simulink library "NCS_Library"  (R2019a)
settings: Solver=VariableStepAuto  StartTime=0.0  StopTime=10.0  RelTol=1e-3
values from neighbouring files (symbols this model uses):
  A = 10    [Parameter.m]
  band = 100000000    [Parameter.m]
  BER = 0    [Parameter.m]
  c = 5000000    [Parameter.m]
  c1 = 4.33    [Parameter.m]
  c2 = 3.16    [Parameter.m]
  CAN2EthernetDelay = 0.000    (= 0)    [Parameter.m]
  cR = 1.5*10^-3    (= 0.0015)    [Parameter.m]
  cw = (cwE * 2 + cwM * (nW_ges-2))/nW_ges    (= 0.1475)    [Parameter.m]
  cwE = 0.35    [Parameter.m]
  cwM = 0.08    [Parameter.m]
  Cycle_Controller = 0    [Parameter.m]
  CyclePLC = 24/1000    (= 0.024)    [Parameter.m]
  d = 800000    [Parameter.m]
  Dr = 0.92    [Parameter.m]
  Ethernet2CANDelay = 0.005    [Parameter.m]
  F_konst = 70892    [Parameter.m]
  FA = 100000    [Parameter.m]
  FB_WB_max = 10000    [Parameter.m]
  FBel_an = iG*nG*F_KZmax*nBan*R_mR/(Dr/2)    (= 28197.4297239)    [Parameter.m]
  FBel_frei = iG*nG*F_KZmax*nBfrei*R_mW/(Dr/2)    (= 29270.6882948)    [Parameter.m]
  Fmaxdyn = 300000    [Parameter.m]
  g = 9.81    [Parameter.m]
  i = 0    [Parameter.m]
  J = 1/2*mA*(Dr/2)^2    (= 158.7)    [Parameter.m]
  k1 = 0.095    [Parameter.m]
  k2 = 9.26/3.6    (= 2.57222222222)    [Parameter.m]
  k3 = 4.63/3.6    (= 1.28611111111)    [Parameter.m]
  mges = 58000    [Parameter.m]
  mu = [mu1 mu2]    [Parameter.m]
  muBel1 = 0.42    [Parameter.m]
  muBel2 = 0.36    [Parameter.m]
  n = 0.001    [Parameter.m]
  n_Mg = 4    [Parameter.m]
  n_WB = 4    [Parameter.m]
  nA = 4    [Parameter.m]
  nBan = 2    [Parameter.m]
  nBfrei = 3    [Parameter.m]
  nM = 4    [Parameter.m]
  nW_an = 4    [Parameter.m]
  P_max = 8200000    [Parameter.m]
  Q = 10    [Parameter.m]
  r_reib = 600    [Parameter.m]
  rho = 1.08    [Parameter.m]
  rhoL = 1.225    [Parameter.m]
  Size = 8    [Parameter.m]
  slip = [s1 s2]    [Parameter.m]
  tol = 0.05    [Parameter.m]
  v00 = 100/3.6    (= 27.7777777778)    [Parameter.m]
  v_grenz = 60/3.6    (= 16.6666666667)    [Parameter.m]
  v_opt = 75/3.6    (= 20.8333333333)    [Parameter.m]
  W_opt = 0.5    [Parameter.m]
  WB = 1    [Parameter.m]
  y_opt = sqrt(W_opt)/((1+sqrt(W_opt))^2+W_opt)    [Parameter.m]
undefined symbols (not defined in the file or in its folder): BUSCapacity, CableLength, controlGate, D_dyn, D_mg, EnableBurst, EnableToF, entity, Entity_out, Gate, Gate_4, Gate_5, Gate_ACK, Gate_copy, Gate_RX, getData, gettime, I_dyn, I_mg, m, magnitude, P_dyn, P_mg, ReadAttributes, readdata, ReadData, ReadSize, sigbuilder_block, Timeout, ToB, ToF, v0, v_d, v_soll
libraries: simulink x176, $bdroot x102
(part 9 of 12)

== system NCS_Library/Network/ETB/Subsystem2/Routing Table/Get Routing Table ==
  note: Compute RT
  note: Receive Data
  note: Send Data
  RouterID : Inport
  s1 : Inport  Port=2
  s2 : Inport  Port=3
  s3 : Inport  Port=4
  Failed : Inport  Port=5
  Compute Routing Table : Subsystem
  Compute routing matrix RM : Subsystem
  Constant1 : Constant
  Constant2 : Constant
  Delay : Delay  DelayLength=1
  Delay1 : Delay  DelayLength=1
  Detect Change : simulink/Logic and Bit Operations/Detect Change  vinit=0  OutDataTypeStr=boolean
  Display : Display
  Entity Gate : EntityGate  InputPortMessageModes=m,m  OutputPortMessageModes=m  OperatingMode=Release gate  OpenGateAtSimulationStart=on
  Entity Generator : EntityGenerator  InputPortMessageModes=m  OutputPortMessageModes=m  GenerationMethod=Event-based  Period=0.5  GenerateAction=[entity.R_local] = writedata();  AttributeName=ID|S1|S2|S3|S4|S5  AttributeInitialValue=1|0|0|0|0|0  EntityType=Bus object  EntityTypeName=Router
      settings: InputPortMap=u0
  Entity Multicast : EntityMulticast  InputPortMessageModes=m  MulticastTag=Router
  Entity Terminator : EntityTerminator  InputPortMessageModes=m  EntryAction=readdata(entity.R_local);  NumberEntitiesArrived=on
      settings: OutputPortMap=o0
  Failed1 : InportShadow  Port=5
  Ground : Ground
  Ground1 : Ground
  Message Send : MessageSend  OutputPortMessageModes=m  ShowEnablePort=on
      settings: InputPortMap=e0,u1
  Message Send1 : MessageSend  OutputPortMessageModes=m  ShowEnablePort=on
      settings: InputPortMap=e0,u1
  Multicast Receive Queue : EntityQueue  OutputPortMessageModes=m  Capacity=50  EntityArrivalSource=Multicast  MulticastTag=Router
      settings: OutputPortMap=o5
  Router Control : Stateflow chart  TreatAsAtomicUnit=on
  RouterID1 : InportShadow
  Simulink Function1 : Subsystem  TreatAsAtomicUnit=on
  Simulink Function2 : Subsystem  TreatAsAtomicUnit=on
  RT : Outport
  FIN : Outport  Port=2
  wires:
  Compute routing matrix RM/2(RM_global) -> Compute Routing Table/2(RM)
  Simulink Function2/1(RM_in) -> Compute routing matrix RM/1(RM_in)
  Compute Routing Table/1(FIN_Init) -> FIN/1, Delay1/1
  RouterID1/1 -> Compute Routing Table/1(ID)
  Message Send/1 -> Entity Gate/1
  Multicast Receive Queue/1 -> Entity Gate/2
  Delay/1 -> Message Send/1
  Detect Change/1 -> Delay/1
  Entity Terminator/1 -> Detect Change/1
  Constant1/1 -> Message Send/2
  Entity Gate/1 -> Entity Terminator/1
  Message Send1/1 -> Entity Generator/1
  Entity Generator/1 -> Entity Multicast/1
  RouterID/1 -> Simulink Function1/1(In1)
  s1/1 -> Simulink Function1/2(s1)
  s2/1 -> Simulink Function1/3(In8)
  s3/1 -> Simulink Function1/4(In9)
  Ground/1 -> Simulink Function1/5(In10)
  Ground1/1 -> Simulink Function1/6(In11)
  Constant2/1 -> Message Send1/2
  Simulink Function2/2(Refresh) -> Router Control/1(Refresh)
  Router Control/2(Init) -> Compute routing matrix RM/Enable
  Router Control/1(Tx) -> Display/1, Message Send1/1
  Compute Routing Table/2(RT) -> RT/1
  Failed/1 -> Simulink Function1/7(Failed)
  Failed1/1 -> Router Control/2(Failed)
  Delay1/1 -> Router Control/3(FIN)
  Compute routing matrix RM/1(FIN_RM) -> Compute Routing Table/Enable

== system NCS_Library/Network/ETB/Subsystem2/Routing Table/Subsystem ==
  Clock : Clock
  Compare To Constant : simulink/Logic and Bit Operations/Compare To Constant  relop=>=  const=ToF  OutDataTypeStr=uint8
  Constant3 : Constant  Value=EnableToF
  Display2 : Display
  Display3 : Display
  Logical Operator : Logic  AllPortsSameDT=off  OutDataTypeStr=boolean
  Out1 : Outport
  wires:
  Compare To Constant/1 -> Logical Operator/1, Display3/1
  Constant3/1 -> Logical Operator/2, Display2/1
  Clock/1 -> Compare To Constant/1
  Logical Operator/1 -> Out1/1

== system NCS_Library/Network/Gateway/Gateway1/CAN Interface/CAN Interface ==
  note: Receiver
  note: Transmitter
  d_in : Inport
  Current Message : EntityQueue  InputPortMessageModes=m  OutputPortMessageModes=m  Capacity=2  EntryAction=controlGate(0);  ExitAction=controlGate(1);
      settings: OutputPortMap=o5
  Damaged Message : EntityTerminator  InputPortMessageModes=m  NumberEntitiesArrived=on
      settings: OutputPortMap=o0
  Display{,1..3} (4 alike) : Display
  Drop Dated Message upon Buffer Overflow : EntityOutputSwitch  InputPortMessageModes=m  OutputPortMessageModes=m,m  SwitchAttributeName=Attribute1
  Entity Replicator : EntityReplicator  InputPortMessageModes=m  OutputPortMessageModes=m,m
  Entity Replicator1 : EntityReplicator  InputPortMessageModes=m  OutputPortMessageModes=m,m
  Entity Terminator : EntityTerminator  InputPortMessageModes=m
  Failure Control CAN : $bdroot/Network/Applications/Failure Control CAN  SystemSampleTime=-1
  Failure Control CAN1 : $bdroot/Network/Applications/Failure Control CAN  SystemSampleTime=-1
  Message Release Control : EntityGate  InputPortMessageModes=m,m  OutputPortMessageModes=m  OpenGateAtSimulationStart=on
  Message from Bus : EntityQueue  OutputPortMessageModes=m  Capacity=20  EntityArrivalSource=Multicast  MulticastTag=FromBus_1
      settings: OutputPortMap=o5
  Path Combiner : EntityInputSwitch  InputPortMessageModes=m,m  OutputPortMessageModes=m
  Re-Transmission Control : Subsystem
  Received Message : EntityServer  InputPortMessageModes=m  OutputPortMessageModes=m  Capacity=1  ServiceTimeValue=0
  Reception Control : Stateflow chart  TreatAsAtomicUnit=on
  Replicate for Re-Transmission : EntityReplicator  InputPortMessageModes=m  OutputPortMessageModes=m,m,m  NumberReplicas=2
      settings: OutputPortMap=o0,o1,o2
  Send Message to Bus : EntityMulticast  InputPortMessageModes=m  MulticastTag=ToBus_1
  Signal To CAN Message : Subsystem
  Simulink Function : Subsystem  TreatAsAtomicUnit=on
  Sort : EntityOutputSwitch  InputPortMessageModes=m,m  OutputPortMessageModes=m,m,m  NumberOutputPorts=3  SwitchingCriterion=From control port  SwitchAttributeName=Attribute1
      settings: InputPortMap=u0,u1  OutputPortMap=o0,o1,o2
  Subscribed Message : EntityTerminator  InputPortMessageModes=m  NumberEntitiesArrived=on
      settings: OutputPortMap=o0
  Transmission Buffer : EntityQueue  InputPortMessageModes=m  OutputPortMessageModes=m  Capacity=15  QueueType=Priority  PrioritySource=ID
      settings: OutputPortMap=o5
  Unsubscribed Message : EntityTerminator  InputPortMessageModes=m  NumberEntitiesArrived=on
      settings: OutputPortMap=o0
  CAN_Message : Outport
  wires:
  Sort/1 -> Entity Replicator1/1
  Failure Control CAN/1 -> Message Release Control/2
  Replicate for Re-Transmission/3 -> Reception Control/1(TX)
  Simulink Function/1(ctrl) -> Message Release Control/1
  Current Message/1 -> Re-Transmission Control/1(IN)
  Reception Control/3(ReTX) -> [ReTX]
  Transmission Buffer/1 -> Failure Control CAN/1
  Re-Transmission Control/1(OUT) -> Drop Dated Message upon Buffer Overflow/1
  Message from Bus/1 -> Failure Control CAN1/1
  Entity Replicator/1 -> Reception Control/2(RX)
  Replicate for Re-Transmission/2 -> Send Message to Bus/1
  Failure Control CAN1/1 -> Entity Replicator/1
  Unsubscribed Message/1 -> Display1/1
  Drop Dated Message upon Buffer Overflow/2 -> Entity Terminator/1
  Path Combiner/1 -> Transmission Buffer/1
  Replicate for Re-Transmission/1 -> Current Message/1
  Damaged Message/1 -> Display/1
  [Reset] -> Re-Transmission Control/3(Reset)
  Re-Transmission Control/2(#TX) -> Display3/1
  d_in/1 -> Signal To CAN Message/1(Data)
  Signal To CAN Message/1(MsgOut) -> Path Combiner/2
  Entity Replicator/2 -> Received Message/1
  Reception Control/2(Success) -> [Reset]
  Drop Dated Message upon Buffer Overflow/1 -> Path Combiner/1
  Subscribed Message/1 -> Display2/1
  [ReTX] -> Re-Transmission Control/2(ReTX)
  Sort/2 -> Unsubscribed Message/1
  Message Release Control/1 -> Replicate for Re-Transmission/1
  Reception Control/1(Port) -> Sort/1
  Sort/3 -> Damaged Message/1
  Received Message/1 -> Sort/2
  Entity Replicator1/2 -> Subscribed Message/1
  Entity Replicator1/1 -> CAN_Message/1

== system NCS_Library/Network/Gateway/Gateway1/CAN Interface/Entry Control ==
  note: new entity in buffer AND buffer is NOT flushed
  note: refresh
  FLUSH : Inport
  n_packets : Inport  Port=2
  Add : Sum
  Add1 : Sum  Inputs=+-
  Compare To Zero : simulink/Logic and Bit Operations/Compare To Zero  relop===  OutDataTypeStr=boolean
  Compare To Zero1 : simulink/Logic and Bit Operations/Compare To Zero  relop=>  OutDataTypeStr=boolean
  Delay : Delay  DelayLength=1  InitialCondition=1
  Display1 : Display
  Enabled Subsystem : Subsystem  TreatAsAtomicUnit=on
  Entity Server : EntityServer  InputPortMessageModes=m  OutputPortMessageModes=n,m  Capacity=1  ServiceTimeValue=0  NumberEntitiesDeparted=on
      settings: OutputPortMap=o0,o9
  FLUSH1 : InportShadow
  Memory : Memory
  Multiply : Product
  Out1 : Outport
  wires:
  n_packets/1 -> Add1/1, Memory/1
  Memory/1 -> Add1/2
  Add1/1 -> Compare To Zero1/1
  Compare To Zero/1 -> Multiply/1
  Compare To Zero1/1 -> Multiply/2
  Multiply/1 -> Add/1
  FLUSH/1 -> Compare To Zero/1
  Add/1 -> Enabled Subsystem/Enable
  Delay/1 -> Add/2
  FLUSH1/1 -> Delay/1
  Entity Server/1 -> Display1/1
  Entity Server/2 -> Out1/1
  Enabled Subsystem/1(Out1) -> Entity Server/1

== system NCS_Library/Network/Gateway/Gateway1/CAN Interface/Gate Control ==
  note: Time condition
  note: Number condition
  n_packets : Inport
  Add : Sum  Inputs=-+
  Add2 : Sum
  Add3 : Sum  Inputs=-+-+
  Clock : Clock
  Compare To Zero : simulink/Logic and Bit Operations/Compare To Zero  relop=>=  OutDataTypeStr=uint8
  Compare To Zero1 : simulink/Logic and Bit Operations/Compare To Zero  relop=>=  OutDataTypeStr=uint8
  Compare To Zero2 : simulink/Logic and Bit Operations/Compare To Zero  relop=>  OutDataTypeStr=uint8
  Constant : Constant  Value=T_Tx
  Constant1 : Constant  Value=MaxNum
  Constant2 : Constant  Value=1e-10
  Memory : Memory  InheritSampleTime=on
  Multiply : Product
  Multiply1 : Product
  Save last release time1 : Subsystem
  FLUSH : Outport
  wires:
  Compare To Zero2/1 -> Multiply/2
  Multiply/1 -> Save last release time1/Enable, FLUSH/1
  Add2/1 -> Multiply/1
  Compare To Zero/1 -> Add2/2
  n_packets/1 -> Add/2, Compare To Zero2/1
  Constant1/1 -> Add/1
  Compare To Zero1/1 -> Add2/1
  Add/1 -> Compare To Zero/1
  Multiply1/1 -> Add3/1
  Constant/1 -> Multiply1/2, Add3/3  "T_Tx"
  Memory/1 -> Multiply1/1, Save last release time1/1(Time)
  Clock/1 -> Add3/2
  Constant2/1 -> Add3/4  "Compensate numeric drift"
  Save last release time1/1(Out1) -> Memory/1
  Add3/1 -> Compare To Zero1/1

== system NCS_Library/Network/Gateway/Gateway1/CAN Interface/Read Data ==
  ReadData : TriggerPort  TriggerType=function-call  IsSimulinkFunction=on  FunctionName=ReadData  FunctionVisibility=scoped  VariantControl=(inherit)
  SensorType : ArgIn  DisableCoverage=on  OutDataTypeStr=uint8  ArgumentName=SensorType
  SensorType1 : ArgIn  DisableCoverage=on  Port=2  ArgumentName=Data
  Type : Outport
  Data : Outport  Port=2  OutputWhenDisabled=reset  InitialOutput=0
  wires:
  SensorType1/1 -> Data/1
  SensorType/1 -> Type/1

== system NCS_Library/Network/Gateway/Gateway1/CAN Interface/Save Data ==
  Type : Inport
  Data : Inport  Port=2
  FLUSH : Inport  Port=3
  Add : Sum
  Delay : Delay  DelayLength=1  InitialCondition=1
  Detect Change : simulink/Logic and Bit Operations/Detect Change  vinit=0  OutDataTypeStr=boolean
  Detect Change1 : simulink/Logic and Bit Operations/Detect Change  vinit=0  OutDataTypeStr=boolean
  Display : Display
  Display1 : Display
  Display2 : Display
  Hold Data : Stateflow chart  TreatAsAtomicUnit=on
  MATLAB Function : MATLAB Function  TreatAsAtomicUnit=on
  Memory : Memory  InheritSampleTime=on
  OutData : Outport
  wires:
  Detect Change1/1 -> Add/2
  Detect Change/1 -> Add/1
  Add/1 -> MATLAB Function/2(write)
  Memory/1 -> MATLAB Function/5(M_Data_old)
  FLUSH/1 -> Hold Data/1(Flush), Delay/1
  MATLAB Function/1(M_Data) -> Hold Data/2(InData), Memory/1
  Type/1 -> Display2/1, MATLAB Function/3(Type), Detect Change/1
  Data/1 -> Display1/1, MATLAB Function/4(Data), Detect Change1/1
  Delay/1 -> MATLAB Function/1(refresh)
  Hold Data/1(OutData) -> OutData/1, Display/1

== system NCS_Library/Network/Gateway/Gateway1/Ethernet Interface/Enabled Subsystem ==
  In1 : Inport
  Enable : EnablePort
  Out1 : Outport
  wires:
  In1/1 -> Out1/1

== system NCS_Library/Network/Gateway/Gateway1/Ethernet Interface/Protocol Stack ==
  Signal : Inport
  Parameter : Inport  Port=2
  RxFromBus : Inport  Port=3
  Bus Creator1 : BusCreator  Inputs=13
  Bus Selector : BusSelector  OutputSignals=SDTv2,T_Tx,msgType
  CycleRx : EntityServer  InputPortMessageModes=m  OutputPortMessageModes=m  Capacity=inf  ServiceTimeValue=CycleRx
  CycleTx : EntityServer  InputPortMessageModes=m  OutputPortMessageModes=m  Capacity=inf  ServiceTimeValue=CycleTx
  Data Type Conversion{,1..6} (7 alike) : DataTypeConversion  OutDataTypeStr=double
  Detect Change : simulink/Logic and Bit Operations/Detect Change  vinit=0  OutDataTypeStr=boolean
  IP : $bdroot/Network/ETB/OSI Layers/IP  SystemSampleTime=-1
  MAC Controller : $bdroot/Network/ETB/OSI Layers/MAC Controller  SystemSampleTime=-1
  Multiply : Product
  SDTv2 : $bdroot/Network/ETB/OSI Layers/SDTv2  SystemSampleTime=-1
  Signal1 : InportShadow
  TRDP PD : $bdroot/Network/ETB/OSI Layers/TRDP PD  SystemSampleTime=-1
  TRDP Timeout : $bdroot/Network/ETB/OSI Layers/TRDP Timeout  SystemSampleTime=-1
  UDP Single-Port : $bdroot/Network/ETB/OSI Layers/UDP Single-Port  SystemSampleTime=-1
  Data : Outport
  Recorder : Outport  Port=2
  TxToBus : Outport  Port=3
  wires:
  Data Type Conversion6/1 -> Bus Creator1/7  "#Receive"
  Data Type Conversion5/1 -> Bus Creator1/9  "#damaged"
  Data Type Conversion4/1 -> Bus Creator1/12  "Retry"
  Data Type Conversion3/1 -> Bus Creator1/3  "SSC"
  Data Type Conversion2/1 -> Bus Creator1/8  "msgType_receive"
  Data Type Conversion1/1 -> Bus Creator1/5  "#Transmit"
  Bus Selector/1 -> SDTv2/2, [SDTv2]  "<SDTv2>"
  Detect Change/1 -> Data Type Conversion4/1
  MAC Controller/3 -> Detect Change/1  "Retry"
  MAC Controller/4 -> TxToBus/1
  Bus Selector/3 -> SDTv2/4  "<msgType>"
  TRDP PD/1 -> SDTv2/5
  Bus Selector/2 -> SDTv2/3  "<T_Tx>"
  TRDP PD/2 -> SDTv2/6
  SDTv2/4 -> TRDP PD/1
  TRDP PD/7 -> UDP Single-Port/1
  Bus Creator1/1 -> Recorder/1
  Data Type Conversion/1 -> Bus Creator1/6  "msgType_transmit"
  Parameter/1 -> TRDP PD/3, MAC Controller/2, IP/2, Bus Selector/1
  Signal/1 -> SDTv2/1, Bus Creator1/1  "Signal"
  MAC Controller/2 -> Bus Creator1/11  "#collision"
  UDP Single-Port/1 -> TRDP PD/4
  IP/1 -> UDP Single-Port/2
  UDP Single-Port/2 -> IP/1
  RxFromBus/1 -> MAC Controller/3
  [SDTv2] -> Bus Creator1/13  "SDTv2"
  SDTv2/2 -> Data Type Conversion3/1
  SDTv2/3 -> Bus Creator1/4  "Phase"
  TRDP PD/3 -> Data Type Conversion1/1
  TRDP PD/4 -> Data Type Conversion/1
  TRDP PD/5 -> TRDP Timeout/1, Data Type Conversion6/1
  TRDP PD/6 -> Data Type Conversion2/1
  IP/2 -> Data Type Conversion5/1
  IP/3 -> Bus Creator1/10  "delay"
  CycleRx/1 -> IP/3
  MAC Controller/1 -> CycleRx/1
  IP/4 -> CycleTx/1
  CycleTx/1 -> MAC Controller/1
  Signal1/1 -> TRDP PD/2  "Signal"
  Multiply/1 -> Data/1, Bus Creator1/2
  SDTv2/1 -> Multiply/2  "Data"
  [Valid] -> Multiply/1
  TRDP Timeout/1 -> [Valid]

== system NCS_Library/Network/Gateway/Gateway1/Ethernet Interface/Subsystem4 ==
  Data : Inport
  Add3 : Sum  Inputs=-+-+
  Chart : Stateflow chart  TreatAsAtomicUnit=on
  Clock : Clock
  Compare To Zero1 : simulink/Logic and Bit Operations/Compare To Zero  relop=>=  OutDataTypeStr=uint8
  Constant8 : Constant  Value=T_Tx_CAN
  Constant9 : Constant  Value=1e-10
  Detect Change : simulink/Logic and Bit Operations/Detect Change  vinit=0  OutDataTypeStr=boolean
  Display : Display
  Display1 : Display
  Display2 : Display
  MATLAB Function : MATLAB Function  TreatAsAtomicUnit=on
  Memory1 : Memory  InheritSampleTime=on
  Multiply1 : Product
  Save num release : Subsystem
  Push : Outport
  wires:
  Add3/1 -> Compare To Zero1/1
  Constant9/1 -> Add3/4  "Compensate numeric drift"
  Save num release/1(Out1) -> Memory1/1
  Constant8/1 -> Multiply1/2, Add3/3  "T_Tx"
  Memory1/1 -> Save num release/1(Time), Multiply1/1
  Multiply1/1 -> Add3/1
  Clock/1 -> Add3/2
  Data/1 -> Display2/1, Detect Change/1, MATLAB Function/1(Data)
  Chart/1(Push) -> Push/1
  Compare To Zero1/1 -> Save num release/Enable, Display1/1, Chart/1(TIME)
  Detect Change/1 -> MATLAB Function/2(Change)
  MATLAB Function/1(NEW) -> Chart/2(NEW), Display/1

== system NCS_Library/Network/Gateway/Gateway1/Ethernet Interface/User Interface ==
  note: User defined Parameters
  Add : Sum  Inputs=+-
  Bus Creator : BusCreator  Inputs=8
  Constant : Constant  Value=Address  OutDataTypeStr=uint16
  Constant1 : Constant  Value=Destination  OutDataTypeStr=uint16
  Constant2 : Constant  Value=0  OutDataTypeStr=double
  Constant3 : Constant  Value=3  OutDataTypeStr=uint8
  Constant4 : Constant  Value=SDTv2  OutDataTypeStr=double
  Constant5 : Constant
  Constant6 : Constant  Value=Port  OutDataTypeStr=uint16
  Constant7 : Constant  Value=ReplyAddress  OutDataTypeStr=uint16
  MATLAB Function : MATLAB Function  TreatAsAtomicUnit=on
  MATLAB Function1 : MATLAB Function  TreatAsAtomicUnit=on
  Subscribe : Constant  Value=Subscribe  OutDataTypeStr=uint16
  Subsystem1 : Subsystem
  Subsystem2 : Subsystem
  Subsystem3 : Subsystem
  Out1 : Outport
  wires:
  Add/1 -> Bus Creator/8  "SDTv2"
  Subscribe/1 -> MATLAB Function1/1(u)
  Constant6/1 -> Bus Creator/5  "Port"
  MATLAB Function1/1(y) -> Bus Creator/3  "Subscribe"
  Constant4/1 -> Add/1
  Constant/1 -> Subsystem1/1(In1)
  Subsystem1/1(Out1) -> Bus Creator/1  "Address"
  Constant3/1 -> MATLAB Function/1(u)
  Subsystem3/1(Out1) -> Bus Creator/4  "ReplyAddress"
  MATLAB Function/1(msgType) -> Bus Creator/7  "msgType"
  Subsystem2/1(Out1) -> Bus Creator/2  "Destination"
  Constant1/1 -> Subsystem2/1(In1)
  Constant2/1 -> Bus Creator/6  "T_Tx"
  Constant5/1 -> Add/2
  Constant7/1 -> Subsystem3/1(In1)
  Bus Creator/1 -> Out1/1

== system NCS_Library/Network/Gateway/Gateway2/CAN Interface/CAN Interface ==
  note: Transmitter
  note: Receiver
  d_in : Inport
  Current Message : EntityQueue  InputPortMessageModes=m  OutputPortMessageModes=m  Capacity=2  EntryAction=controlGate(0);  ExitAction=controlGate(1);
      settings: OutputPortMap=o5
  Damaged Message : EntityTerminator  InputPortMessageModes=m  NumberEntitiesArrived=on
      settings: OutputPortMap=o0
  Display{,1..3} (4 alike) : Display
  Drop Dated Message upon Buffer Overflow : EntityOutputSwitch  InputPortMessageModes=m  OutputPortMessageModes=m,m  SwitchAttributeName=Attribute1
  Entity Replicator : EntityReplicator  InputPortMessageModes=m  OutputPortMessageModes=m,m
  Entity Replicator1 : EntityReplicator  InputPortMessageModes=m  OutputPortMessageModes=m,m
  Entity Terminator : EntityTerminator  InputPortMessageModes=m
  Failure Control CAN : $bdroot/Network/Applications/Failure Control CAN  SystemSampleTime=-1
  Failure Control CAN1 : $bdroot/Network/Applications/Failure Control CAN  SystemSampleTime=-1
  Message Release Control : EntityGate  InputPortMessageModes=m,m  OutputPortMessageModes=m  OpenGateAtSimulationStart=on
  Message from Bus : EntityQueue  OutputPortMessageModes=m  Capacity=20  EntityArrivalSource=Multicast  MulticastTag=FromBus_2
      settings: OutputPortMap=o5
  Path Combiner : EntityInputSwitch  InputPortMessageModes=m,m  OutputPortMessageModes=m
  Re-Transmission Control : Subsystem
  Received Message : EntityServer  InputPortMessageModes=m  OutputPortMessageModes=m  Capacity=1  ServiceTimeValue=0
  Reception Control : Stateflow chart  TreatAsAtomicUnit=on
  Replicate for Re-Transmission : EntityReplicator  InputPortMessageModes=m  OutputPortMessageModes=m,m,m  NumberReplicas=2
      settings: OutputPortMap=o0,o1,o2
  Send Message to Bus : EntityMulticast  InputPortMessageModes=m  MulticastTag=ToBus_2
  Signal To CAN Message : Subsystem
  Simulink Function : Subsystem  TreatAsAtomicUnit=on
  Sort : EntityOutputSwitch  InputPortMessageModes=m,m  OutputPortMessageModes=m,m,m  NumberOutputPorts=3  SwitchingCriterion=From control port  SwitchAttributeName=Attribute1
      settings: InputPortMap=u0,u1  OutputPortMap=o0,o1,o2
  Subscribed Message : EntityTerminator  InputPortMessageModes=m  NumberEntitiesArrived=on
      settings: OutputPortMap=o0
  Transmission Buffer : EntityQueue  InputPortMessageModes=m  OutputPortMessageModes=m  Capacity=15  QueueType=Priority  PrioritySource=ID
      settings: OutputPortMap=o5
  Unsubscribed Message : EntityTerminator  InputPortMessageModes=m  NumberEntitiesArrived=on
      settings: OutputPortMap=o0
  CAN_Message : Outport
  wires:
  Entity Replicator1/1 -> CAN_Message/1
  Entity Replicator1/2 -> Subscribed Message/1
  Received Message/1 -> Sort/2
  Sort/3 -> Damaged Message/1
  Reception Control/1(Port) -> Sort/1
  Message Release Control/1 -> Replicate for Re-Transmission/1
  Sort/2 -> Unsubscribed Message/1
  [ReTX] -> Re-Transmission Control/2(ReTX)
  Subscribed Message/1 -> Display2/1
  Drop Dated Message upon Buffer Overflow/1 -> Path Combiner/1
  Reception Control/2(Success) -> [Reset]
  Entity Replicator/2 -> Received Message/1
  Signal To CAN Message/1(MsgOut) -> Path Combiner/2
  d_in/1 -> Signal To CAN Message/1(Data)
  Re-Transmission Control/2(#TX) -> Display3/1
  [Reset] -> Re-Transmission Control/3(Reset)
  Damaged Message/1 -> Display/1
  Replicate for Re-Transmission/1 -> Current Message/1
  Path Combiner/1 -> Transmission Buffer/1
  Drop Dated Message upon Buffer Overflow/2 -> Entity Terminator/1
  Unsubscribed Message/1 -> Display1/1
  Failure Control CAN1/1 -> Entity Replicator/1
  Replicate for Re-Transmission/2 -> Send Message to Bus/1
  Entity Replicator/1 -> Reception Control/2(RX)
  Message from Bus/1 -> Failure Control CAN1/1
  Re-Transmission Control/1(OUT) -> Drop Dated Message upon Buffer Overflow/1
  Transmission Buffer/1 -> Failure Control CAN/1
  Reception Control/3(ReTX) -> [ReTX]
  Current Message/1 -> Re-Transmission Control/1(IN)
  Simulink Function/1(ctrl) -> Message Release Control/1
  Replicate for Re-Transmission/3 -> Reception Control/1(TX)
  Failure Control CAN/1 -> Message Release Control/2
  Sort/1 -> Entity Replicator1/1

== system NCS_Library/Network/Gateway/Gateway2/CAN Interface/Entry Control ==
  note: refresh
  note: new entity in buffer AND buffer is NOT flushed
  FLUSH : Inport
  n_packets : Inport  Port=2
  Add : Sum
  Add1 : Sum  Inputs=+-
  Compare To Zero : simulink/Logic and Bit Operations/Compare To Zero  relop===  OutDataTypeStr=boolean
  Compare To Zero1 : simulink/Logic and Bit Operations/Compare To Zero  relop=>  OutDataTypeStr=boolean
  Delay : Delay  DelayLength=1  InitialCondition=1
  Display1 : Display
  Enabled Subsystem : Subsystem  TreatAsAtomicUnit=on
  Entity Server : EntityServer  InputPortMessageModes=m  OutputPortMessageModes=n,m  Capacity=1  ServiceTimeValue=0  NumberEntitiesDeparted=on
      settings: OutputPortMap=o0,o9
  FLUSH1 : InportShadow
  Memory : Memory
  Multiply : Product
  Out1 : Outport
  wires:
  Enabled Subsystem/1(Out1) -> Entity Server/1
  Entity Server/2 -> Out1/1
  Entity Server/1 -> Display1/1
  FLUSH1/1 -> Delay/1
  Delay/1 -> Add/2
  Add/1 -> Enabled Subsystem/Enable
  FLUSH/1 -> Compare To Zero/1
  Multiply/1 -> Add/1
  Compare To Zero1/1 -> Multiply/2
  Compare To Zero/1 -> Multiply/1
  Add1/1 -> Compare To Zero1/1
  Memory/1 -> Add1/2
  n_packets/1 -> Memory/1, Add1/1

== system NCS_Library/Network/Gateway/Gateway2/CAN Interface/Gate Control ==
  note: Number condition
  note: Time condition
  n_packets : Inport
  Add : Sum  Inputs=-+
  Add2 : Sum
  Add3 : Sum  Inputs=-+-+
  Clock : Clock
  Compare To Zero : simulink/Logic and Bit Operations/Compare To Zero  relop=>=  OutDataTypeStr=uint8
  Compare To Zero1 : simulink/Logic and Bit Operations/Compare To Zero  relop=>=  OutDataTypeStr=uint8
  Compare To Zero2 : simulink/Logic and Bit Operations/Compare To Zero  relop=>  OutDataTypeStr=uint8
  Constant : Constant  Value=T_Tx
  Constant1 : Constant  Value=MaxNum
  Constant2 : Constant  Value=1e-10
  Memory : Memory  InheritSampleTime=on
  Multiply : Product
  Multiply1 : Product
  Save last release time1 : Subsystem
  FLUSH : Outport
  wires:
  Add3/1 -> Compare To Zero1/1
  Save last release time1/1(Out1) -> Memory/1
  Constant2/1 -> Add3/4  "Compensate numeric drift"
  Clock/1 -> Add3/2
  Memory/1 -> Save last release time1/1(Time), Multiply1/1
  Constant/1 -> Add3/3, Multiply1/2  "T_Tx"
  Multiply1/1 -> Add3/1
  Add/1 -> Compare To Zero/1
  Compare To Zero1/1 -> Add2/1
  Constant1/1 -> Add/1
  n_packets/1 -> Compare To Zero2/1, Add/2
  Compare To Zero/1 -> Add2/2
  Add2/1 -> Multiply/1
  Multiply/1 -> FLUSH/1, Save last release time1/Enable
  Compare To Zero2/1 -> Multiply/2

== system NCS_Library/Network/Gateway/Gateway2/CAN Interface/Read Data ==
  ReadData : TriggerPort  TriggerType=function-call  IsSimulinkFunction=on  FunctionName=ReadData  FunctionVisibility=scoped  VariantControl=(inherit)
  SensorType : ArgIn  DisableCoverage=on  OutDataTypeStr=uint8  ArgumentName=SensorType
  SensorType1 : ArgIn  DisableCoverage=on  Port=2  ArgumentName=Data
  Type : Outport
  Data : Outport  Port=2  OutputWhenDisabled=reset  InitialOutput=0
  wires:
  SensorType/1 -> Type/1
  SensorType1/1 -> Data/1

== system NCS_Library/Network/Gateway/Gateway2/CAN Interface/Save Data ==
  Type : Inport
  Data : Inport  Port=2
  FLUSH : Inport  Port=3
  Add : Sum
  Delay : Delay  DelayLength=1  InitialCondition=1
  Detect Change : simulink/Logic and Bit Operations/Detect Change  vinit=0  OutDataTypeStr=boolean
  Detect Change1 : simulink/Logic and Bit Operations/Detect Change  vinit=0  OutDataTypeStr=boolean
  Display : Display
  Display1 : Display
  Display2 : Display
  Hold Data : Stateflow chart  TreatAsAtomicUnit=on
  MATLAB Function : MATLAB Function  TreatAsAtomicUnit=on
  Memory : Memory  InheritSampleTime=on
  OutData : Outport
  wires:
  Hold Data/1(OutData) -> Display/1, OutData/1
  Delay/1 -> MATLAB Function/1(refresh)
  Data/1 -> Detect Change1/1, MATLAB Function/4(Data), Display1/1
  Type/1 -> Detect Change/1, MATLAB Function/3(Type), Display2/1
  MATLAB Function/1(M_Data) -> Memory/1, Hold Data/2(InData)
  FLUSH/1 -> Delay/1, Hold Data/1(Flush)
  Memory/1 -> MATLAB Function/5(M_Data_old)
  Add/1 -> MATLAB Function/2(write)
  Detect Change/1 -> Add/1
  Detect Change1/1 -> Add/2

== system NCS_Library/Network/Gateway/Gateway2/Ethernet Interface/Enabled Subsystem ==
  In1 : Inport
  Enable : EnablePort
  Out1 : Outport
  wires:
  In1/1 -> Out1/1

== system NCS_Library/Network/Gateway/Gateway2/Ethernet Interface/Subsystem ==
  Signal : Inport
  Parameter : Inport  Port=2
  RxFromBus : Inport  Port=3
  Bus Creator1 : BusCreator  Inputs=13
  Bus Selector : BusSelector  OutputSignals=SDTv2,T_Tx,msgType
  CycleRx : EntityServer  InputPortMessageModes=m  OutputPortMessageModes=m  Capacity=inf  ServiceTimeValue=CycleRx
  CycleTx : EntityServer  InputPortMessageModes=m  OutputPortMessageModes=m  Capacity=inf  ServiceTimeValue=CycleTx
  Data Type Conversion{,1..6} (7 alike) : DataTypeConversion  OutDataTypeStr=double
  Detect Change : simulink/Logic and Bit Operations/Detect Change  vinit=0  OutDataTypeStr=boolean
  IP : $bdroot/Network/ETB/OSI Layers/IP  SystemSampleTime=-1
  MAC Controller : $bdroot/Network/ETB/OSI Layers/MAC Controller  SystemSampleTime=-1
  Multiply : Product
  SDTv2 : $bdroot/Network/ETB/OSI Layers/SDTv2  SystemSampleTime=-1
  Signal1 : InportShadow
  TRDP PD : $bdroot/Network/ETB/OSI Layers/TRDP PD  SystemSampleTime=-1
  TRDP Timeout : $bdroot/Network/ETB/OSI Layers/TRDP Timeout  SystemSampleTime=-1
  UDP Single-Port : $bdroot/Network/ETB/OSI Layers/UDP Single-Port  SystemSampleTime=-1
  Data : Outport
  Recorder : Outport  Port=2
  TxToBus : Outport  Port=3
  wires:
  TRDP Timeout/1 -> [Valid]
  [Valid] -> Multiply/1
  SDTv2/1 -> Multiply/2  "Data"
  Multiply/1 -> Bus Creator1/2, Data/1
  Signal1/1 -> TRDP PD/2  "Signal"
  CycleTx/1 -> MAC Controller/1
  IP/4 -> CycleTx/1
  MAC Controller/1 -> CycleRx/1
  CycleRx/1 -> IP/3
  IP/3 -> Bus Creator1/10  "delay"
  IP/2 -> Data Type Conversion5/1
  TRDP PD/6 -> Data Type Conversion2/1
  TRDP PD/5 -> Data Type Conversion6/1, TRDP Timeout/1
  TRDP PD/4 -> Data Type Conversion/1
  TRDP PD/3 -> Data Type Conversion1/1
  SDTv2/3 -> Bus Creator1/4  "Phase"
  SDTv2/2 -> Data Type Conversion3/1
  [SDTv2] -> Bus Creator1/13  "SDTv2"
  RxFromBus/1 -> MAC Controller/3
  UDP Single-Port/2 -> IP/1
  IP/1 -> UDP Single-Port/2
  UDP Single-Port/1 -> TRDP PD/4
  MAC Controller/2 -> Bus Creator1/11  "#collision"
  Signal/1 -> Bus Creator1/1, SDTv2/1  "Signal"
  Parameter/1 -> Bus Selector/1, IP/2, MAC Controller/2, TRDP PD/3
  Data Type Conversion/1 -> Bus Creator1/6  "msgType_transmit"
  Bus Creator1/1 -> Recorder/1
  TRDP PD/7 -> UDP Single-Port/1
  SDTv2/4 -> TRDP PD/1
  TRDP PD/2 -> SDTv2/6
  Bus Selector/2 -> SDTv2/3  "<T_Tx>"
  TRDP PD/1 -> SDTv2/5
  Bus Selector/3 -> SDTv2/4  "<msgType>"
  MAC Controller/4 -> TxToBus/1
  MAC Controller/3 -> Detect Change/1  "Retry"
  Detect Change/1 -> Data Type Conversion4/1
  Bus Selector/1 -> [SDTv2], SDTv2/2  "<SDTv2>"
  Data Type Conversion1/1 -> Bus Creator1/5  "#Transmit"
  Data Type Conversion2/1 -> Bus Creator1/8  "msgType_receive"
  Data Type Conversion3/1 -> Bus Creator1/3  "SSC"
  Data Type Conversion4/1 -> Bus Creator1/12  "Retry"
  Data Type Conversion5/1 -> Bus Creator1/9  "#damaged"
  Data Type Conversion6/1 -> Bus Creator1/7  "#Receive"

== system NCS_Library/Network/Gateway/Gateway2/Ethernet Interface/Subsystem1 ==
  In1 : Inport
  Constant : Constant  Value=0  OutDataTypeStr=uint16
  Constant1 : Constant  Value=0  OutDataTypeStr=uint16
  Mux : Mux  Inputs=3
  Out1 : Outport
  wires:
  Constant1/1 -> Mux/3
  Constant/1 -> Mux/2
  Mux/1 -> Out1/1
  In1/1 -> Mux/1

== system NCS_Library/Network/Gateway/Gateway2/Ethernet Interface/Subsystem2 ==
  In1 : Inport
  Constant : Constant  Value=0  OutDataTypeStr=uint16
  Constant1 : Constant  Value=0  OutDataTypeStr=uint16
  Mux : Mux  Inputs=3
  Out1 : Outport
  wires:
  In1/1 -> Mux/1
  Mux/1 -> Out1/1
  Constant/1 -> Mux/2
  Constant1/1 -> Mux/3

== system NCS_Library/Network/Gateway/Gateway2/Ethernet Interface/Subsystem3 ==
  In1 : Inport
  Constant : Constant  Value=0  OutDataTypeStr=uint16
  Constant1 : Constant  Value=0  OutDataTypeStr=uint16
  Mux : Mux  Inputs=3
  Out1 : Outport
  wires:
  Constant1/1 -> Mux/3
  Constant/1 -> Mux/2
  Mux/1 -> Out1/1
  In1/1 -> Mux/1

== system NCS_Library/Network/Gateway/Gateway2/Ethernet Interface/Subsystem4 ==
  Data : Inport
  Add3 : Sum  Inputs=-+-+
  Chart : Stateflow chart  TreatAsAtomicUnit=on
  Clock : Clock
  Compare To Zero1 : simulink/Logic and Bit Operations/Compare To Zero  relop=>=  OutDataTypeStr=uint8
  Constant8 : Constant  Value=T_Tx_CAN
  Constant9 : Constant  Value=1e-10
  Detect Change : simulink/Logic and Bit Operations/Detect Change  vinit=0  OutDataTypeStr=boolean
  Display : Display
  Display2 : Display
  MATLAB Function : MATLAB Function  TreatAsAtomicUnit=on
  Memory1 : Memory  InheritSampleTime=on
  Multiply1 : Product
  Save num release : Subsystem
  Push : Outport
  wires:
  MATLAB Function/1(NEW) -> Chart/2(NEW), Display/1
  Detect Change/1 -> MATLAB Function/2(Change)
  Compare To Zero1/1 -> Chart/1(TIME), Save num release/Enable
  Chart/1(Push) -> Push/1
  Data/1 -> MATLAB Function/1(Data), Detect Change/1, Display2/1
  Clock/1 -> Add3/2
  Multiply1/1 -> Add3/1
  Memory1/1 -> Multiply1/1, Save num release/1(Time)
  Constant8/1 -> Add3/3, Multiply1/2  "T_Tx"
  Save num release/1(Out1) -> Memory1/1
  Constant9/1 -> Add3/4  "Compensate numeric drift"
  Add3/1 -> Compare To Zero1/1

== system NCS_Library/Plant (Train)/angetriebener Endwagen Merz/Achse_1/Bremskraft pro angetriebener Achse1/Belagreibwert_Nennwerte ==
  v : Inport
  Add : Sum
  Add1 : Sum
  Compare To Constant : simulink/Logic and Bit Operations/Compare To Constant  relop=<=  const=200/3.6  OutDataTypeStr=boolean
  Compare To Constant3 : simulink/Logic and Bit Operations/Compare To Constant  relop=>  const=200/3.6  OutDataTypeStr=boolean
  Compare To Constant4 : simulink/Logic and Bit Operations/Compare To Constant  relop=>=  const=0  OutDataTypeStr=boolean
  Constant1 : Constant  Value=muBel1
  Constant6 : Constant  Value=muBel1-muBel2
  Gain1 : Gain  Gain=3.6/100
  Gain2 : Gain  Gain=2
  Product1 : Product  Inputs=3
  Product3 : Product
  Product4 : Product
  Subtract1 : Sum  Inputs=+-
  mühBel : Outport
  wires:
  Compare To Constant/1 -> Product1/3
  Constant1/1 -> Add1/1, Product1/2
  Compare To Constant3/1 -> Product3/1
  v/1 -> Compare To Constant4/1, Product4/2, Compare To Constant3/1, Compare To Constant/1
  Add1/1 -> Subtract1/1
  Constant6/1 -> Gain2/1, Gain1/1
  Gain1/1 -> Product4/1
  Product4/1 -> Subtract1/2
  Subtract1/1 -> Product3/2
  Product1/1 -> Add/1
  Product3/1 -> Add/2
  Add/1 -> mühBel/1
  Compare To Constant4/1 -> Product1/1
  Gain2/1 -> Add1/2

== system NCS_Library/Plant (Train)/angetriebener Endwagen Merz/Achse_1/Bremskraft pro angetriebener Achse1/max dynamische Bremse pro angetriebener Achse ==
  v : Inport
  Add : Sum  Inputs=+++
  Add1 : Sum
  Compare To Constant : simulink/Logic and Bit Operations/Compare To Constant  relop=<=  const=29  OutDataTypeStr=boolean
  Compare To Constant1 : simulink/Logic and Bit Operations/Compare To Constant  relop=>  const=29  OutDataTypeStr=boolean
  Compare To Constant2 : simulink/Logic and Bit Operations/Compare To Constant  relop=>  const=4.2  OutDataTypeStr=boolean
  Compare To Constant3 : simulink/Logic and Bit Operations/Compare To Constant  relop=<=  const=4.2  OutDataTypeStr=boolean
  Divide : Product  Inputs=*/
  Fmax : Constant  Value=Fmaxdyn
  Fmax1 : Constant  Value=F_konst
  Gain : Gain  Gain=r_reib
  Gain1 : Gain  Gain=1/(nA*nW_an)
  Leistung : Constant  Value=P_max
  Logical Operator : Logic  AllPortsSameDT=off  OutDataTypeStr=boolean
  Product : Product
  Product1 : Product
  Product2 : Product  Inputs=3
  Subtract : Sum  Inputs=+-
  Um Fehler zu vermeiden : Constant  Value=0.001
  FB : Outport
  wires:
  Leistung/1 -> Divide/1
  Fmax/1 -> Subtract/1
  Gain/1 -> Subtract/2
  Subtract/1 -> Product/1
  Compare To Constant/1 -> Logical Operator/1
  Product/1 -> Add/2
  Add/1 -> Gain1/1
  Divide/1 -> Product1/1
  Product1/1 -> Add/3
  Gain1/1 -> FB/1
  Compare To Constant1/1 -> Product1/2
  v/1 -> Add1/1, Compare To Constant1/1, Product2/2, Compare To Constant3/1, Compare To Constant2/1, Gain/1, Compare To Constant/1
  Um Fehler zu vermeiden/1 -> Add1/2
  Logical Operator/1 -> Product/2
  Compare To Constant2/1 -> Logical Operator/2
  Fmax1/1 -> Product2/1
  Compare To Constant3/1 -> Product2/3
  Product2/1 -> Add/1
  Add1/1 -> Divide/2

== system NCS_Library/Plant (Train)/angetriebener Endwagen Merz/Achse_2/Bremskraft pro angetriebener Achse2/Belagreibwert_Nennwerte ==
  v : Inport
  Add : Sum
  Add1 : Sum
  Compare To Constant : simulink/Logic and Bit Operations/Compare To Constant  relop=<=  const=200/3.6  OutDataTypeStr=boolean
  Compare To Constant3 : simulink/Logic and Bit Operations/Compare To Constant  relop=>  const=200/3.6  OutDataTypeStr=boolean
  Compare To Constant4 : simulink/Logic and Bit Operations/Compare To Constant  relop=>=  const=0  OutDataTypeStr=boolean
  Constant1 : Constant  Value=muBel1
  Constant6 : Constant  Value=muBel1-muBel2
  Gain1 : Gain  Gain=3.6/100
  Gain2 : Gain  Gain=2
  Product1 : Product  Inputs=3
  Product3 : Product
  Product4 : Product
  Subtract1 : Sum  Inputs=+-
  mühBel : Outport
  wires:
  Compare To Constant/1 -> Product1/3
  Constant1/1 -> Add1/1, Product1/2
  Compare To Constant3/1 -> Product3/1
  v/1 -> Compare To Constant4/1, Product4/2, Compare To Constant3/1, Compare To Constant/1
  Add1/1 -> Subtract1/1
  Constant6/1 -> Gain2/1, Gain1/1
  Gain1/1 -> Product4/1
  Product4/1 -> Subtract1/2
  Subtract1/1 -> Product3/2
  Product1/1 -> Add/1
  Product3/1 -> Add/2
  Add/1 -> mühBel/1
  Compare To Constant4/1 -> Product1/1
  Gain2/1 -> Add1/2

== system NCS_Library/Plant (Train)/angetriebener Endwagen Merz/Achse_2/Bremskraft pro angetriebener Achse2/max dynamische Bremse pro angetriebener Achse ==
  v : Inport
  Add : Sum  Inputs=+++
  Add1 : Sum
  Compare To Constant : simulink/Logic and Bit Operations/Compare To Constant  relop=<=  const=29  OutDataTypeStr=boolean
  Compare To Constant1 : simulink/Logic and Bit Operations/Compare To Constant  relop=>  const=29  OutDataTypeStr=boolean
  Compare To Constant2 : simulink/Logic and Bit Operations/Compare To Constant  relop=>  const=4.2  OutDataTypeStr=boolean
  Compare To Constant3 : simulink/Logic and Bit Operations/Compare To Constant  relop=<=  const=4.2  OutDataTypeStr=boolean
  Divide : Product  Inputs=*/
  Fmax : Constant  Value=Fmaxdyn
  Fmax1 : Constant  Value=F_konst
  Gain : Gain  Gain=r_reib
  Gain1 : Gain  Gain=1/(nA*nW_an)
  Leistung : Constant  Value=P_max
  Logical Operator : Logic  AllPortsSameDT=off  OutDataTypeStr=boolean
  Product : Product
  Product1 : Product
  Product2 : Product  Inputs=3
  Subtract : Sum  Inputs=+-
  Um Fehler zu vermeiden : Constant  Value=0.001
  FB : Outport
  wires:
  Leistung/1 -> Divide/1
  Fmax/1 -> Subtract/1
  Gain/1 -> Subtract/2
  Subtract/1 -> Product/1
  Compare To Constant/1 -> Logical Operator/1
  Product/1 -> Add/2
  Add/1 -> Gain1/1
  Divide/1 -> Product1/1
  Product1/1 -> Add/3
  Gain1/1 -> FB/1
  Compare To Constant1/1 -> Product1/2
  v/1 -> Add1/1, Compare To Constant1/1, Product2/2, Compare To Constant3/1, Compare To Constant2/1, Gain/1, Compare To Constant/1
  Um Fehler zu vermeiden/1 -> Add1/2
  Logical Operator/1 -> Product/2
  Compare To Constant2/1 -> Logical Operator/2
  Fmax1/1 -> Product2/1
  Compare To Constant3/1 -> Product2/3
  Product2/1 -> Add/1
  Add1/1 -> Divide/2

== system NCS_Library/Plant (Train)/angetriebener Endwagen Merz/Achse_3/Bremskraft pro angetriebener Achse3/Belagreibwert_Nennwerte ==
  v : Inport
  Add : Sum
  Add1 : Sum
  Compare To Constant : simulink/Logic and Bit Operations/Compare To Constant  relop=<=  const=200/3.6  OutDataTypeStr=boolean
  Compare To Constant3 : simulink/Logic and Bit Operations/Compare To Constant  relop=>  const=200/3.6  OutDataTypeStr=boolean
  Compare To Constant4 : simulink/Logic and Bit Operations/Compare To Constant  relop=>=  const=0  OutDataTypeStr=boolean
  Constant1 : Constant  Value=muBel1
  Constant6 : Constant  Value=muBel1-muBel2
  Gain1 : Gain  Gain=3.6/100
  Gain2 : Gain  Gain=2
  Product1 : Product  Inputs=3
  Product3 : Product
  Product4 : Product
  Subtract1 : Sum  Inputs=+-
  mühBel : Outport
  wires:
  Compare To Constant/1 -> Product1/3
  Constant1/1 -> Add1/1, Product1/2
  Compare To Constant3/1 -> Product3/1
  v/1 -> Compare To Constant4/1, Product4/2, Compare To Constant3/1, Compare To Constant/1
  Add1/1 -> Subtract1/1
  Constant6/1 -> Gain2/1, Gain1/1
  Gain1/1 -> Product4/1
  Product4/1 -> Subtract1/2
  Subtract1/1 -> Product3/2
  Product1/1 -> Add/1
  Product3/1 -> Add/2
  Add/1 -> mühBel/1
  Compare To Constant4/1 -> Product1/1
  Gain2/1 -> Add1/2

== system NCS_Library/Plant (Train)/angetriebener Endwagen Merz/Achse_3/Bremskraft pro angetriebener Achse3/max dynamische Bremse pro angetriebener Achse ==
  v : Inport
  Add : Sum  Inputs=+++
  Add1 : Sum
  Compare To Constant : simulink/Logic and Bit Operations/Compare To Constant  relop=<=  const=29  OutDataTypeStr=boolean
  Compare To Constant1 : simulink/Logic and Bit Operations/Compare To Constant  relop=>  const=29  OutDataTypeStr=boolean
  Compare To Constant2 : simulink/Logic and Bit Operations/Compare To Constant  relop=>  const=4.2  OutDataTypeStr=boolean
  Compare To Constant3 : simulink/Logic and Bit Operations/Compare To Constant  relop=<=  const=4.2  OutDataTypeStr=boolean
  Divide : Product  Inputs=*/
  Fmax : Constant  Value=Fmaxdyn
  Fmax1 : Constant  Value=F_konst
  Gain : Gain  Gain=r_reib
  Gain1 : Gain  Gain=1/(nA*nW_an)
  Leistung : Constant  Value=P_max
  Logical Operator : Logic  AllPortsSameDT=off  OutDataTypeStr=boolean
  Product : Product
  Product1 : Product
  Product2 : Product  Inputs=3
  Subtract : Sum  Inputs=+-
  Um Fehler zu vermeiden : Constant  Value=0.001
  FB : Outport
  wires:
  Leistung/1 -> Divide/1
  Fmax/1 -> Subtract/1
  Gain/1 -> Subtract/2
  Subtract/1 -> Product/1
  Compare To Constant/1 -> Logical Operator/1
  Product/1 -> Add/2
  Add/1 -> Gain1/1
  Divide/1 -> Product1/1
  Product1/1 -> Add/3
  Gain1/1 -> FB/1
  Compare To Constant1/1 -> Product1/2
  v/1 -> Add1/1, Compare To Constant1/1, Product2/2, Compare To Constant3/1, Compare To Constant2/1, Gain/1, Compare To Constant/1
  Um Fehler zu vermeiden/1 -> Add1/2
  Logical Operator/1 -> Product/2
  Compare To Constant2/1 -> Logical Operator/2
  Fmax1/1 -> Product2/1
  Compare To Constant3/1 -> Product2/3
  Product2/1 -> Add/1
  Add1/1 -> Divide/2

== system NCS_Library/Plant (Train)/angetriebener Endwagen Merz/Achse_4/Bremskraft pro angetriebener Achse4/Belagreibwert_Nennwerte ==
  v : Inport
  Add : Sum
  Add1 : Sum
  Compare To Constant : simulink/Logic and Bit Operations/Compare To Constant  relop=<=  const=200/3.6  OutDataTypeStr=boolean
  Compare To Constant3 : simulink/Logic and Bit Operations/Compare To Constant  relop=>  const=200/3.6  OutDataTypeStr=boolean
  Compare To Constant4 : simulink/Logic and Bit Operations/Compare To Constant  relop=>=  const=0  OutDataTypeStr=boolean
  Constant1 : Constant  Value=muBel1
  Constant6 : Constant  Value=muBel1-muBel2
  Gain1 : Gain  Gain=3.6/100
  Gain2 : Gain  Gain=2
  Product1 : Product  Inputs=3
  Product3 : Product
  Product4 : Product
  Subtract1 : Sum  Inputs=+-
  mühBel : Outport
  wires:
  Compare To Constant/1 -> Product1/3
  Constant1/1 -> Add1/1, Product1/2
  Compare To Constant3/1 -> Product3/1
  v/1 -> Compare To Constant4/1, Product4/2, Compare To Constant3/1, Compare To Constant/1
  Add1/1 -> Subtract1/1
  Constant6/1 -> Gain2/1, Gain1/1
  Gain1/1 -> Product4/1
  Product4/1 -> Subtract1/2
  Subtract1/1 -> Product3/2
  Product1/1 -> Add/1
  Product3/1 -> Add/2
  Add/1 -> mühBel/1
  Compare To Constant4/1 -> Product1/1
  Gain2/1 -> Add1/2

== system NCS_Library/Plant (Train)/angetriebener Endwagen Merz/Achse_4/Bremskraft pro angetriebener Achse4/max dynamische Bremse pro angetriebener Achse ==
  v : Inport
  Add : Sum  Inputs=+++
  Add1 : Sum
  Compare To Constant : simulink/Logic and Bit Operations/Compare To Constant  relop=<=  const=29  OutDataTypeStr=boolean
  Compare To Constant1 : simulink/Logic and Bit Operations/Compare To Constant  relop=>  const=29  OutDataTypeStr=boolean
  Compare To Constant2 : simulink/Logic and Bit Operations/Compare To Constant  relop=>  const=4.2  OutDataTypeStr=boolean
  Compare To Constant3 : simulink/Logic and Bit Operations/Compare To Constant  relop=<=  const=4.2  OutDataTypeStr=boolean
  Divide : Product  Inputs=*/
  Fmax : Constant  Value=Fmaxdyn
  Fmax1 : Constant  Value=F_konst
  Gain : Gain  Gain=r_reib
  Gain1 : Gain  Gain=1/(nA*nW_an)
  Leistung : Constant  Value=P_max
  Logical Operator : Logic  AllPortsSameDT=off  OutDataTypeStr=boolean
  Product : Product
  Product1 : Product
  Product2 : Product  Inputs=3
  Subtract : Sum  Inputs=+-
  Um Fehler zu vermeiden : Constant  Value=0.001
  FB : Outport
  wires:
  Leistung/1 -> Divide/1
  Fmax/1 -> Subtract/1
  Gain/1 -> Subtract/2
  Subtract/1 -> Product/1
  Compare To Constant/1 -> Logical Operator/1
  Product/1 -> Add/2
  Add/1 -> Gain1/1
  Divide/1 -> Product1/1
  Product1/1 -> Add/3
  Gain1/1 -> FB/1
  Compare To Constant1/1 -> Product1/2
  v/1 -> Add1/1, Compare To Constant1/1, Product2/2, Compare To Constant3/1, Compare To Constant2/1, Gain/1, Compare To Constant/1
  Um Fehler zu vermeiden/1 -> Add1/2
  Logical Operator/1 -> Product/2
  Compare To Constant2/1 -> Logical Operator/2
  Fmax1/1 -> Product2/1
  Compare To Constant3/1 -> Product2/3
  Product2/1 -> Add/1
  Add1/1 -> Divide/2

== system NCS_Library/Plant (Train)/freier Wagen/Bremskraft Schienenbremse/WB Bremse pro Wagen/Subsystem ==
  v : Inport
  Add : Sum
  Add1 : Sum
  Berechnung W : Subsystem
  Compare To Zero : simulink/Logic and Bit Operations/Compare To Zero  relop=>=  OutDataTypeStr=boolean
  Constant : Constant
  Divide : Product  Inputs=*/
  Math Function : Math  Operator=magnitude^2  SaturateOnIntegerOverflow=on
  Product : Product
  Sqrt : Sqrt  SaturateOnIntegerOverflow=on
  y : Outport
  wires:
  v/1 -> Berechnung W/1(v)
  Product/1 -> Add1/2, Sqrt/1
  Sqrt/1 -> Add/1, Divide/1
  Constant/1 -> Add/2
  Add/1 -> Math Function/1
  Math Function/1 -> Add1/1
  Divide/1 -> y/1
  Add1/1 -> Divide/2
  Berechnung W/1(W) -> Compare To Zero/1, Product/2
  Compare To Zero/1 -> Product/1

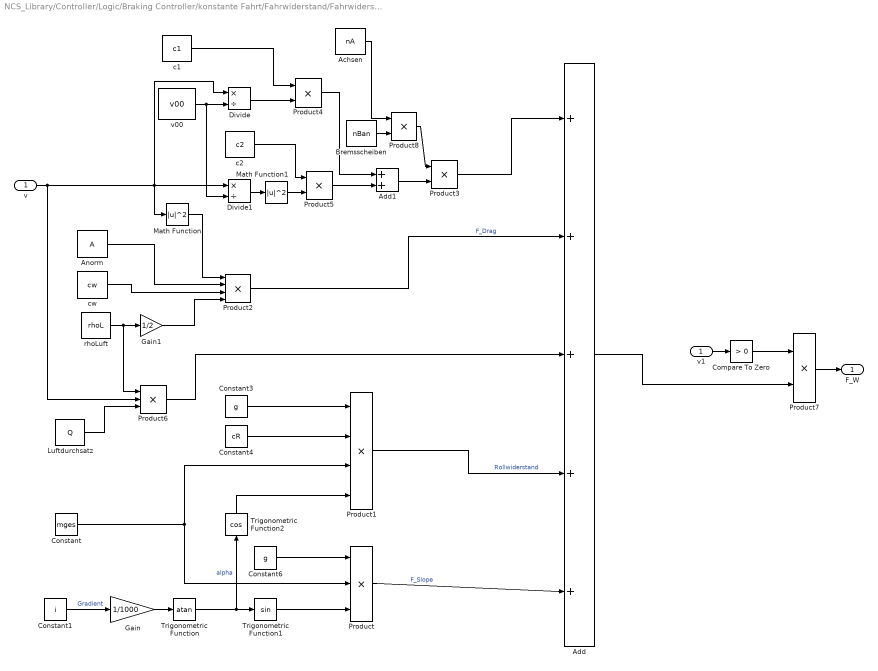
== system NCS_Library/Controller/Logic/Braking Controller/konstante Fahrt/Fahrwiderstand/Fahrwiderstand_angeWagen ==
  v : Inport
  Achsen : Constant  Value=nA
  Add : Sum  Inputs=+++++
  Add1 : Sum
  Anorm : Constant  Value=A
  Bremsscheiben : Constant  Value=nBan
  Compare To Zero : simulink/Logic and Bit Operations/Compare To Zero  relop=>  OutDataTypeStr=boolean
  Constant : Constant  Value=mges
  Constant1 : Constant  Value=i
  Constant3 : Constant  Value=g
  Constant4 : Constant  Value=cR
  Constant6 : Constant  Value=g
  Divide : Product  Inputs=*/
  Divide1 : Product  Inputs=*/
  Gain : Gain  Gain=1/1000
  Gain1 : Gain  Gain=1/2
  Luftdurchsatz : Constant  Value=Q
  Math Function : Math  Operator=magnitude^2  SaturateOnIntegerOverflow=on
  Math Function1 : Math  Operator=magnitude^2  SaturateOnIntegerOverflow=on
  Product : Product  Inputs=3
  Product1 : Product  Inputs=4
  Product2 : Product  Inputs=4
  Product{3..5,7..8} (5 alike) : Product
  Product6 : Product  Inputs=3
  Trigonometric Function : Trigonometry  Operator=atan
  Trigonometric Function1 : Trigonometry
  Trigonometric Function2 : Trigonometry  Operator=cos
  c1 : Constant  Value=c1
  c2 : Constant  Value=c2
  cw : Constant  Value=cw
  rhoLuft : Constant  Value=rhoL
  v00 : Constant  Value=v00
  v1 : InportShadow
  F_W : Outport
  wires:
  Trigonometric Function2/1 -> Product1/4
  Bremsscheiben/1 -> Product8/2
  Product8/1 -> Product3/1
  Compare To Zero/1 -> Product7/1
  Product7/1 -> F_W/1
  Math Function1/1 -> Product5/2
  Product6/1 -> Add/3
  Luftdurchsatz/1 -> Product6/3
  c2/1 -> Product5/1
  Math Function/1 -> Product2/1
  Divide1/1 -> Math Function1/1
  Product5/1 -> Add1/2
  Product4/1 -> Add1/1
  Divide/1 -> Product4/2
  v00/1 -> Divide/2, Divide1/2
  c1/1 -> Product4/1
  Add1/1 -> Product3/2
  Product3/1 -> Add/1
  Achsen/1 -> Product8/1
  Product2/1 -> Add/2  "F_Drag"
  Gain1/1 -> Product2/4
  cw/1 -> Product2/3
  Anorm/1 -> Product2/2
  v/1 -> Math Function/1, Divide/1, Divide1/1, Product6/2
  rhoLuft/1 -> Gain1/1, Product6/1
  Product1/1 -> Add/4  "Rollwiderstand"
  Constant/1 -> Product/2, Product1/3
  Constant4/1 -> Product1/2
  Constant3/1 -> Product1/1
  Add/1 -> Product7/2
  Product/1 -> Add/5  "F_Slope"
  Trigonometric Function1/1 -> Product/3
  Constant6/1 -> Product/1
  Gain/1 -> Trigonometric Function/1
  Trigonometric Function/1 -> Trigonometric Function1/1, Trigonometric Function2/1  "alpha"
  Constant1/1 -> Gain/1  "Gradient"
  v1/1 -> Compare To Zero/1
